simulink model "Hiv_tunet_vs_ikketunet"  (R2022a)
settings: Solver=VariableStepAuto  StartTime=0.0  StopTime=15  RelTol=1e-3
values from neighbouring files (symbols this model uses):
  A_topp = 0.286615    [Modell_verdier.m]
  C_D = 1.28    [Modell_verdier.m]
  g = 9.81    [Modell_verdier.m]
  masse = 22.49    [Modell_verdier.m]
  tetthet_vann = 1000    [Modell_verdier.m]
libraries: spsFirstOrderFilterLib x2
settings Model: Creator=andre  LastModifiedBy=andre

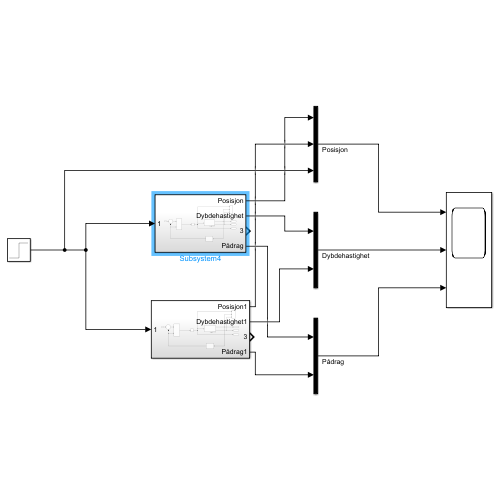
[thumbnail: Simulink's stored preview of the top-level diagram]
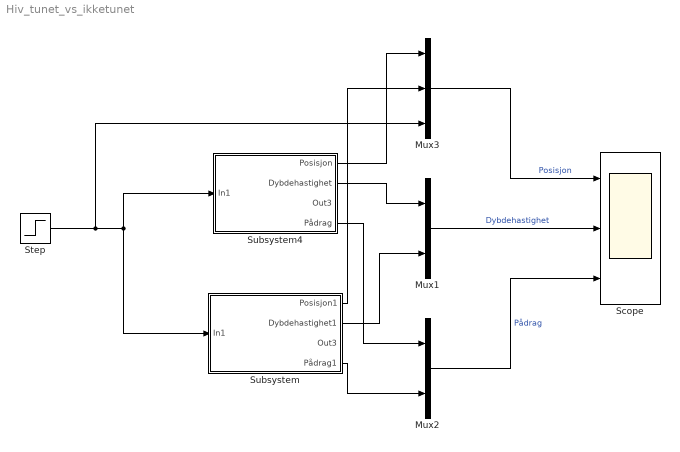
== system Hiv_tunet_vs_ikketunet ==
  Mux1 : Mux  Inputs=2
  Mux2 : Mux  Inputs=2
  Mux3 : Mux  Inputs=3
  Scope : Scope  NumInputPorts=3
  Step : Step  After=0.4  SampleTime=0
  Subsystem : Subsystem
  Subsystem4 : Subsystem
  wires:
  Step/1 -> Mux3/3, Subsystem4/1(In1), Subsystem/1(In1)
  Subsystem/4(Pådrag1) -> Mux2/2
  Subsystem4/4(Pådrag) -> Mux2/1
  Mux2/1 -> Scope/3  "Pådrag"
  Subsystem/2(Dybdehastighet1) -> Mux1/2
  Mux1/1 -> Scope/2  "Dybdehastighet"
  Subsystem/1(Posisjon1) -> Mux3/2
  Subsystem4/1(Posisjon) -> Mux3/1
  Mux3/1 -> Scope/1  "Posisjon"
  Subsystem4/2(Dybdehastighet) -> Mux1/1

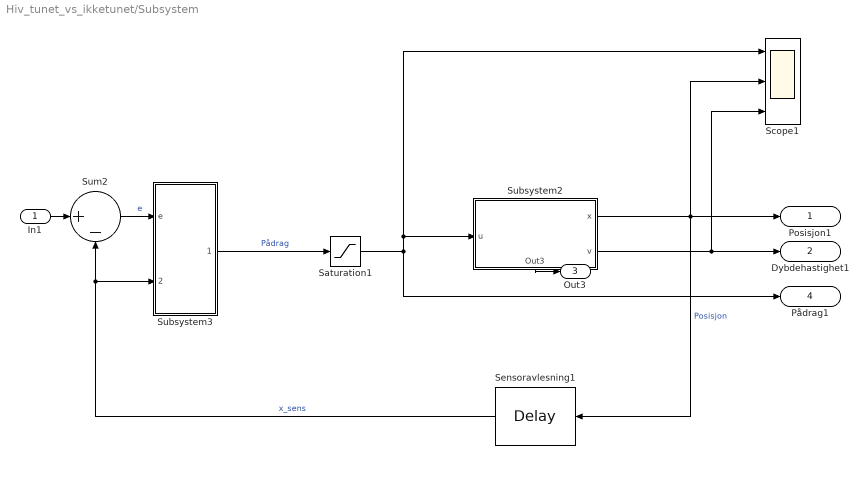
== system Hiv_tunet_vs_ikketunet/Subsystem ==
  In1 : Inport
  Saturation1 : Saturate  UpperLimit=2.8  LowerLimit=-2.8
  Scope1 : Scope  NumInputPorts=3
  Sensoravlesning1 : TransportDelay  DelayTime=0.2
  Subsystem2 : Subsystem
      settings: PortSchema="{\"entries\":[{\"content\":{\"sides\":[{\"content\":{\"connectorIds\":[\"In1\"]},\"type\":\"ConnectorPlacement.EquallySpacedRectSide\",\"uuid\":\"a8a29be1-14bc-435c-85b5-ac35e3907c96\"},{\"content\":{\"connectorIds\":[\"Out1\",\"Out2\"],\"side\":\"RIGHT\"},\"type\":\"ConnectorPlacement.EquallySpacedRectSide\",\"uuid\":\"5af08fbc-e738-4b37-b103-fc6d4045b140\"},{\"content\":{\"connectorIds\":[],\"side\":\"TOP\"},\"type\":\"ConnectorPlacement.EquallySpacedRectSide\",\"uuid\":\"224b0456-6b51-420d-ad14-0122555d3363\"},{\"content\":{\"connectorIds\":[\"Out3\"],\"side\":\"BOTTOM\"},\"type\":\"ConnectorPlacement.EquallySpacedRectSide\",\"uuid\":\"0b4c62fc-fd11-42a7-809f-bd90d82071b6\"}]},\"type\":\"ConnectorPlacement.EquallySpacedConnector\",\"uuid\":\"7d1a238c-0f98-4fb6-8cfc-e343dda97f61\"}],\"packageUris\":[\"http://schema.mathworks.com/mf0/Connector/R2020b\"],\"version\":\"1.0\"}"
  Subsystem3 : Subsystem
  Sum2 : Sum  Inputs=|+-
  Posisjon1 : Outport
  Dybdehastighet1 : Outport  Port=2
  Out3 : Outport  Port=3
  Pådrag1 : Outport  Port=4
  wires:
  Subsystem2/2(v) -> Dybdehastighet1/1, Scope1/3
  Saturation1/1 -> Pådrag1/1, Scope1/1, Subsystem2/1(u)
  Sum2/1 -> Subsystem3/1(e)  "e"
  Sensoravlesning1/1 -> Sum2/2, Subsystem3/2(y_sensor)  "x_sens"
  In1/1 -> Sum2/1
  Subsystem2/1(x) -> Posisjon1/1, Sensoravlesning1/1, Scope1/2  "Posisjon"
  Subsystem2/3(Out3) -> Out3/1
  Subsystem3/1(Pådrag) -> Saturation1/1  "Pådrag"

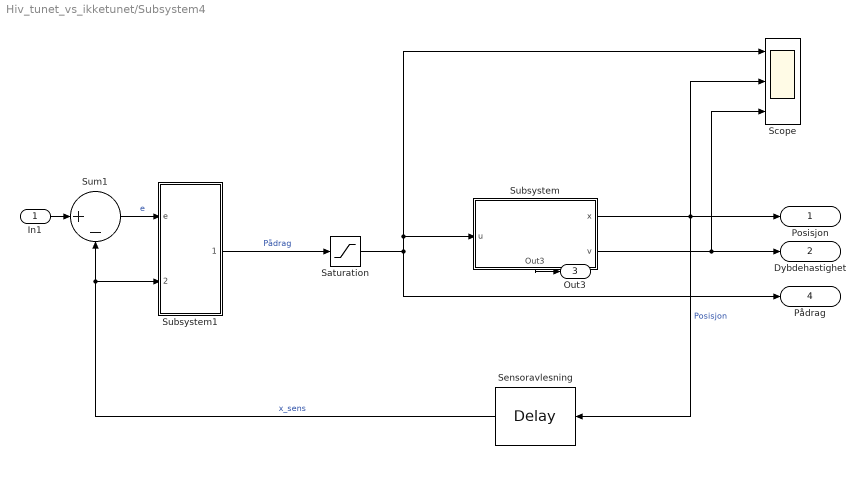
== system Hiv_tunet_vs_ikketunet/Subsystem4 ==
  In1 : Inport
  Saturation : Saturate  UpperLimit=2.8  LowerLimit=-2.8
  Scope : Scope  NumInputPorts=3
  Sensoravlesning : TransportDelay  DelayTime=0.2
  Subsystem : Subsystem
      settings: PortSchema="{\"entries\":[{\"content\":{\"sides\":[{\"content\":{\"connectorIds\":[\"In1\"]},\"type\":\"ConnectorPlacement.EquallySpacedRectSide\",\"uuid\":\"a8a29be1-14bc-435c-85b5-ac35e3907c96\"},{\"content\":{\"connectorIds\":[\"Out1\",\"Out2\"],\"side\":\"RIGHT\"},\"type\":\"ConnectorPlacement.EquallySpacedRectSide\",\"uuid\":\"5af08fbc-e738-4b37-b103-fc6d4045b140\"},{\"content\":{\"connectorIds\":[],\"side\":\"TOP\"},\"type\":\"ConnectorPlacement.EquallySpacedRectSide\",\"uuid\":\"224b0456-6b51-420d-ad14-0122555d3363\"},{\"content\":{\"connectorIds\":[\"Out3\"],\"side\":\"BOTTOM\"},\"type\":\"ConnectorPlacement.EquallySpacedRectSide\",\"uuid\":\"0b4c62fc-fd11-42a7-809f-bd90d82071b6\"}]},\"type\":\"ConnectorPlacement.EquallySpacedConnector\",\"uuid\":\"7d1a238c-0f98-4fb6-8cfc-e343dda97f61\"}],\"packageUris\":[\"http://schema.mathworks.com/mf0/Connector/R2020b\"],\"version\":\"1.0\"}"
  Subsystem1 : Subsystem
  Sum1 : Sum  Inputs=|+-
  Posisjon : Outport
  Dybdehastighet : Outport  Port=2
  Out3 : Outport  Port=3
  Pådrag : Outport  Port=4
  wires:
  Sum1/1 -> Subsystem1/1(e)  "e"
  Sensoravlesning/1 -> Sum1/2, Subsystem1/2(y_sensor)  "x_sens"
  Saturation/1 -> Pådrag/1, Scope/1, Subsystem/1(u)
  In1/1 -> Sum1/1
  Subsystem/2(v) -> Dybdehastighet/1, Scope/3
  Subsystem1/1(Pådrag) -> Saturation/1  "Pådrag"
  Subsystem/3(Out3) -> Out3/1
  Subsystem/1(x) -> Posisjon/1, Sensoravlesning/1, Scope/2  "Posisjon"

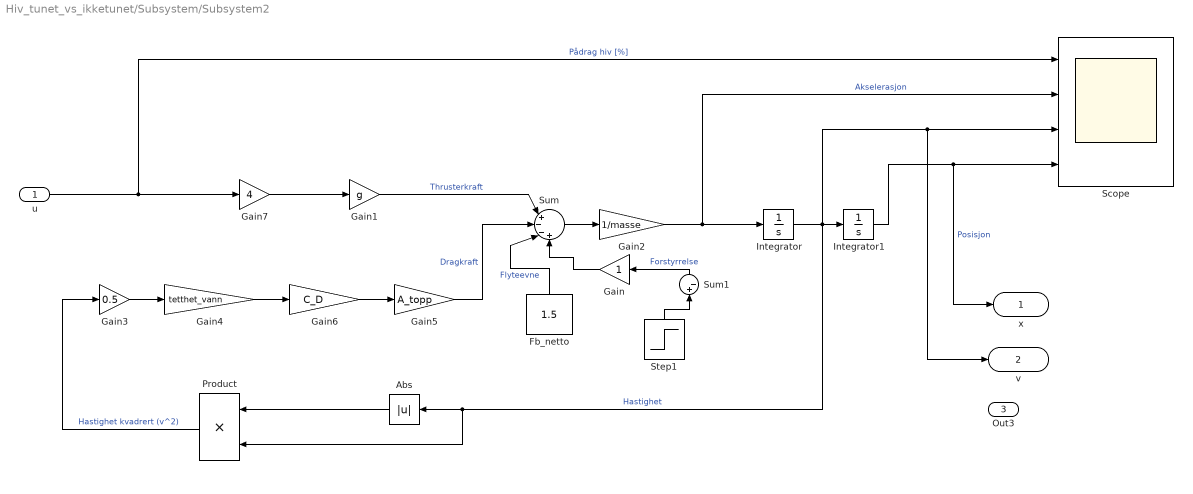
== system Hiv_tunet_vs_ikketunet/Subsystem/Subsystem2 ==
  u : Inport
  Abs : Abs  SaturateOnIntegerOverflow=off
  Fb_netto : Constant  Value=1.5
  Gain : Gain
  Gain1 : Gain  Gain=g
  Gain2 : Gain  Gain=1/masse
  Gain3 : Gain  Gain=0.5
  Gain4 : Gain  Gain=tetthet_vann
  Gain5 : Gain  Gain=A_topp
  Gain6 : Gain  Gain=C_D
  Gain7 : Gain  Gain=4
  Integrator : Integrator  InitialCondition=0.1
  Integrator1 : Integrator
  Product : Product
  Scope : Scope  NumInputPorts=4
  Step1 : Step  Time=7  After=35  SampleTime=0
  Sum : Sum  Inputs=|+--+
  Sum1 : Sum  Inputs=|+-
  x : Outport
  v : Outport  Port=2
  Out3 : Outport  Port=3
  wires:
  Gain6/1 -> Gain5/1
  Integrator1/1 -> x/1, Scope/4  "Posisjon"
  Gain5/1 -> Sum/2  "Dragkraft"
  Gain2/1 -> Integrator/1, Scope/2  "Akselerasjon"
  Gain1/1 -> Sum/1  "Thrusterkraft"
  Gain4/1 -> Gain6/1
  Gain3/1 -> Gain4/1
  Fb_netto/1 -> Sum/3  "Flyteevne"
  Integrator/1 -> Integrator1/1, Product/2, Abs/1, v/1, Scope/3  "Hastighet"
  Product/1 -> Gain3/1  "Hastighet kvadrert (v^2)"
  u/1 -> Gain7/1, Scope/1  "Pådrag hiv [%]"
  Abs/1 -> Product/1
  Sum/1 -> Gain2/1
  Gain7/1 -> Gain1/1
  Gain/1 -> Sum/4
  Sum1/1 -> Gain/1  "Forstyrrelse"
  Step1/1 -> Sum1/1

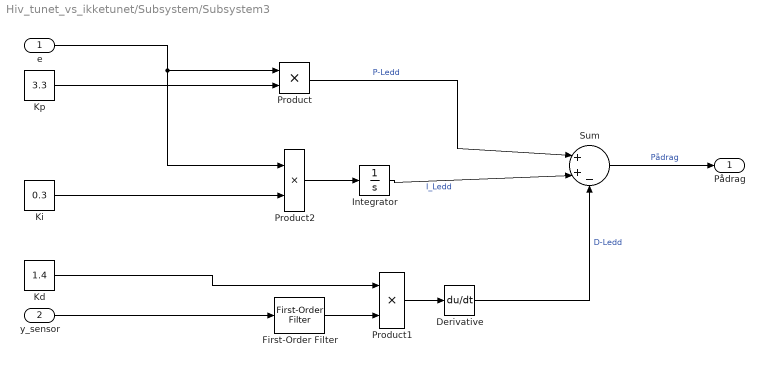
== system Hiv_tunet_vs_ikketunet/Subsystem/Subsystem3 ==
  e : Inport
  y_sensor : Inport  Port=2
  Derivative : Derivative
  First-Order Filter : spsFirstOrderFilterLib/First-Order Filter  FilterType=Lowpass  Tc=(1.451)*0.05  Ts=0  Initialize=on  Vac_Init=[0, 0, 60]  Vdc_Init=0  PlotResponse=off  FreqRange="[0,  200,  1]"
  Integrator : Integrator  LimitOutput=on  UpperSaturationLimit=0.3  LowerSaturationLimit=-0.3
  Kd : Constant  Value=1.4
  Ki : Constant  Value=0.3
  Kp : Constant  Value=3.3
  Product : Product
  Product1 : Product
  Product2 : Product
  Sum : Sum  Inputs=|++-
  Pådrag : Outport
  wires:
  Product2/1 -> Integrator/1
  Kp/1 -> Product/2
  Product/1 -> Sum/1  "P-Ledd"
  y_sensor/1 -> First-Order Filter/1
  Kd/1 -> Product1/1
  e/1 -> Product/1, Product2/1
  Ki/1 -> Product2/2
  First-Order Filter/1 -> Product1/2
  Integrator/1 -> Sum/2  "I_Ledd"
  Sum/1 -> Pådrag/1  "Pådrag"
  Product1/1 -> Derivative/1
  Derivative/1 -> Sum/3  "D-Ledd"

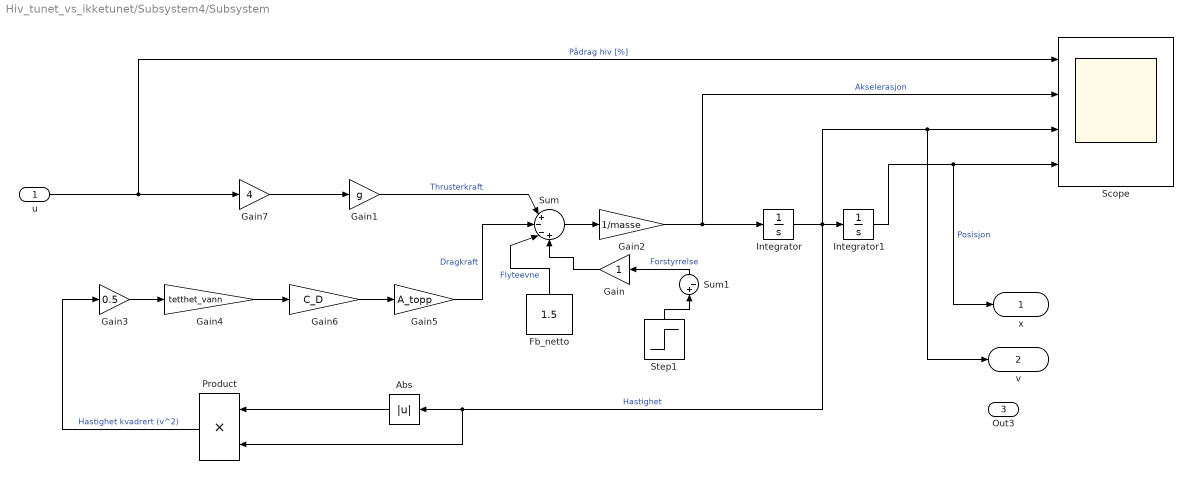
== system Hiv_tunet_vs_ikketunet/Subsystem4/Subsystem ==
  u : Inport
  Abs : Abs  SaturateOnIntegerOverflow=off
  Fb_netto : Constant  Value=1.5
  Gain : Gain
  Gain1 : Gain  Gain=g
  Gain2 : Gain  Gain=1/masse
  Gain3 : Gain  Gain=0.5
  Gain4 : Gain  Gain=tetthet_vann
  Gain5 : Gain  Gain=A_topp
  Gain6 : Gain  Gain=C_D
  Gain7 : Gain  Gain=4
  Integrator : Integrator  InitialCondition=0.1
  Integrator1 : Integrator
  Product : Product
  Scope : Scope  NumInputPorts=4
  Step1 : Step  Time=7  After=35  SampleTime=0
  Sum : Sum  Inputs=|+--+
  Sum1 : Sum  Inputs=|+-
  x : Outport
  v : Outport  Port=2
  Out3 : Outport  Port=3
  wires:
  Gain6/1 -> Gain5/1
  Integrator1/1 -> x/1, Scope/4  "Posisjon"
  Gain5/1 -> Sum/2  "Dragkraft"
  Gain2/1 -> Integrator/1, Scope/2  "Akselerasjon"
  Gain1/1 -> Sum/1  "Thrusterkraft"
  Gain4/1 -> Gain6/1
  Gain3/1 -> Gain4/1
  Fb_netto/1 -> Sum/3  "Flyteevne"
  Integrator/1 -> Integrator1/1, Product/2, Abs/1, v/1, Scope/3  "Hastighet"
  Product/1 -> Gain3/1  "Hastighet kvadrert (v^2)"
  u/1 -> Gain7/1, Scope/1  "Pådrag hiv [%]"
  Abs/1 -> Product/1
  Sum/1 -> Gain2/1
  Gain7/1 -> Gain1/1
  Gain/1 -> Sum/4
  Sum1/1 -> Gain/1  "Forstyrrelse"
  Step1/1 -> Sum1/1

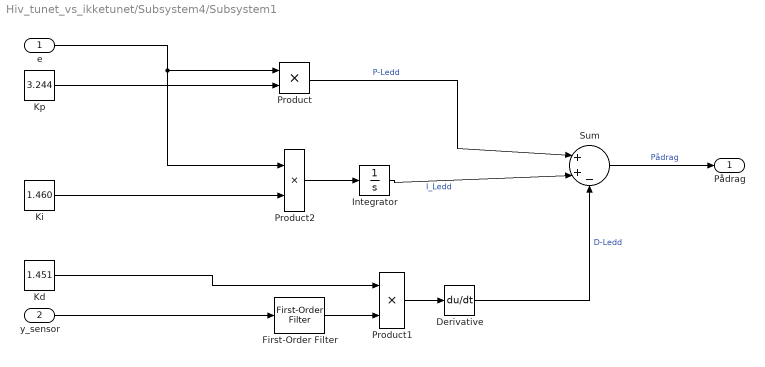
== system Hiv_tunet_vs_ikketunet/Subsystem4/Subsystem1 ==
  e : Inport
  y_sensor : Inport  Port=2
  Derivative : Derivative
  First-Order Filter : spsFirstOrderFilterLib/First-Order Filter  FilterType=Lowpass  Tc=(1.451)*0.05  Ts=0  Initialize=on  Vac_Init=[0, 0, 60]  Vdc_Init=0  PlotResponse=off  FreqRange="[0,  200,  1]"
  Integrator : Integrator  LimitOutput=on  UpperSaturationLimit=0.3  LowerSaturationLimit=-0.3
  Kd : Constant  Value=1.451
  Ki : Constant  Value=1.460
  Kp : Constant  Value=3.244
  Product : Product
  Product1 : Product
  Product2 : Product
  Sum : Sum  Inputs=|++-
  Pådrag : Outport
  wires:
  Product2/1 -> Integrator/1
  Kp/1 -> Product/2
  Product/1 -> Sum/1  "P-Ledd"
  y_sensor/1 -> First-Order Filter/1
  Kd/1 -> Product1/1
  e/1 -> Product/1, Product2/1
  Ki/1 -> Product2/2
  First-Order Filter/1 -> Product1/2
  Integrator/1 -> Sum/2  "I_Ledd"
  Sum/1 -> Pådrag/1  "Pådrag"
  Product1/1 -> Derivative/1
  Derivative/1 -> Sum/3  "D-Ledd"
